simulink model "part1"  (R2021a)
settings: Solver=FixedStepDiscrete  StartTime=0  StopTime=20  FixedStep=0.1  RelTol=1e-3
values from neighbouring files (symbols this model uses):
  mu = [-2.06408447904 -1.49508472185]    [dataSet.mat]
  sig = [50.3880002876 29.2458553231]    [dataSet.mat]
undefined symbols (not defined in the file or in its folder): egoTargetSpd_kph
libraries: deeplib x2, fuzblock x1
settings Model: Creator=Ally  LastModifiedBy=Ally

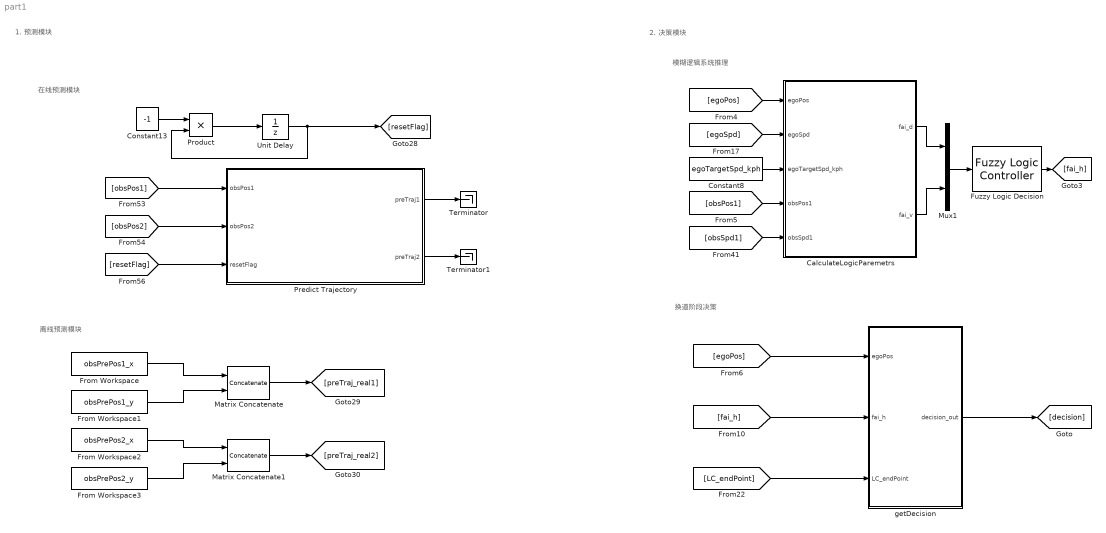
== system part1 ==
  note: 换道阶段决策
  note: 模糊逻辑系统推理
  note: 在线预测模块
  note: 离线预测模块
  note: 2. 决策模块
  note: 1. 预测模块
  CalculateLogicParemetrs : MATLAB Function  TreatAsAtomicUnit=on
  Constant13 : Constant  Value=-1
  Constant8 : Constant  Value=egoTargetSpd_kph
  From Workspace : FromWorkspace  VariableName=obsPrePos1_x
  From Workspace1 : FromWorkspace  VariableName=obsPrePos1_y
  From Workspace2 : FromWorkspace  VariableName=obsPrePos2_x
  From Workspace3 : FromWorkspace  VariableName=obsPrePos2_y
  Fuzzy Logic Decision : fuzblock/Fuzzy Logic  Controller  FIS='LCD.fis'  OutputSampleNumber=101  DataType=double  FuzzifiedInputs=off  RuleFiringStrengths=off  RuleOutputs=off  AggregatedOutputs=off  SimulateUsing=Interpreted execution  OutOfRangeInputValueMessage=warning  NoRuleFiredMessage=warning  EmptyOutputFuzzySetMessage=warning
  Matrix Concatenate : Concatenate  Mode=Multidimensional array  ConcatenateDimension=2
  Matrix Concatenate1 : Concatenate  Mode=Multidimensional array  ConcatenateDimension=2
  Mux1 : Mux  Inputs=2
  Predict Trajectory : Subsystem  TreatAsAtomicUnit=on
  Product : Product
  Terminator : Terminator
  Terminator1 : Terminator
  Unit Delay : UnitDelay  InitialCondition=1  SampleTime=-1  HasFrameUpgradeWarning=on
  getDecision : MATLAB Function  TreatAsAtomicUnit=on
  wires:
  CalculateLogicParemetrs/1(fai_d) -> Mux1/1
  [egoPos] -> CalculateLogicParemetrs/1(egoPos)
  getDecision/1(decision_out) -> [decision]
  CalculateLogicParemetrs/2(fai_v) -> Mux1/2
  [egoSpd] -> CalculateLogicParemetrs/2(egoSpd)
  [LC_endPoint] -> getDecision/3(LC_endPoint)
  Mux1/1 -> Fuzzy Logic Decision/1
  [egoPos] -> getDecision/1(egoPos)
  Constant8/1 -> CalculateLogicParemetrs/3(egoTargetSpd_kph)
  [obsPos1] -> CalculateLogicParemetrs/4(obsPos1)
  [obsSpd1] -> CalculateLogicParemetrs/5(obsSpd1)
  Product/1 -> Unit Delay/1
  Unit Delay/1 -> [resetFlag], Product/2
  Constant13/1 -> Product/1
  [resetFlag] -> Predict Trajectory/3(resetFlag)
  [obsPos1] -> Predict Trajectory/1(obsPos1)
  [obsPos2] -> Predict Trajectory/2(obsPos2)
  Predict Trajectory/1(preTraj1) -> Terminator/1
  Predict Trajectory/2(preTraj2) -> Terminator1/1
  From Workspace/1 -> Matrix Concatenate/1
  From Workspace1/1 -> Matrix Concatenate/2
  From Workspace2/1 -> Matrix Concatenate1/1
  From Workspace3/1 -> Matrix Concatenate1/2
  Matrix Concatenate/1 -> [preTraj_real1]
  Matrix Concatenate1/1 -> [preTraj_real2]
  Fuzzy Logic Decision/1 -> [fai_h]
  [fai_h] -> getDecision/2(fai_h)

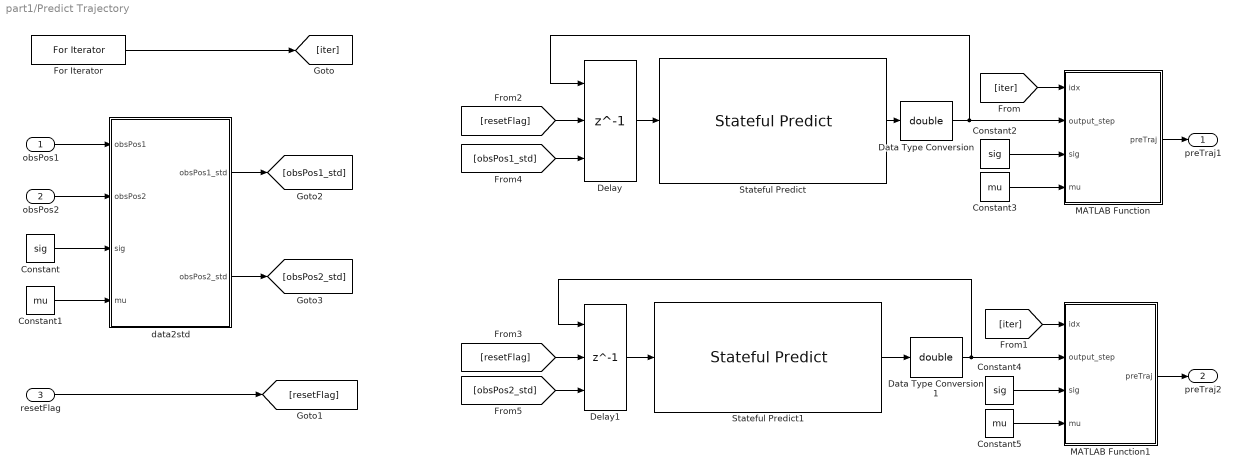
== system part1/Predict Trajectory ==
  obsPos1 : Inport
  obsPos2 : Inport  Port=2
  resetFlag : Inport  Port=3
  Constant : Constant  Value=sig
  Constant1 : Constant  Value=mu
  Constant2 : Constant  Value=sig
  Constant3 : Constant  Value=mu
  Constant4 : Constant  Value=sig
  Constant5 : Constant  Value=mu
  Data Type Conversion : DataTypeConversion  OutDataTypeStr=double
  Data Type Conversion1 : DataTypeConversion  OutDataTypeStr=double
  Delay : Delay  DelayLength=1  InitialConditionSource=Input port  ExternalReset=Either
      settings: InputPortMap=u0,r5,p4
  Delay1 : Delay  DelayLength=1  InitialConditionSource=Input port  ExternalReset=Either
      settings: InputPortMap=u0,r5,p4
  For Iterator : ForIterator  IterationLimit=80
  MATLAB Function : MATLAB Function  TreatAsAtomicUnit=on
  MATLAB Function1 : MATLAB Function  TreatAsAtomicUnit=on
  Stateful Predict : deeplib/Stateful Predict  Network=Network from MAT-file  NetworkFunction=untitled  NetworkFilePath=C:\Users\Ally\Desktop\LSTM.mat  InputDataFormats={ '', '' }  SampleTime=-1  ForceInterpretedSim=off  EnableDLNetwork=on
      settings: SourceProductBaseCode=NN
  Stateful Predict1 : deeplib/Stateful Predict  Network=Network from MAT-file  NetworkFunction=untitled  NetworkFilePath=C:\Users\Ally\Desktop\LSTM.mat  InputDataFormats={ '', '' }  SampleTime=-1  ForceInterpretedSim=off  EnableDLNetwork=on
      settings: SourceProductBaseCode=NN
  data2std : MATLAB Function  TreatAsAtomicUnit=on
  preTraj1 : Outport
  preTraj2 : Outport  Port=2
  wires:
  Delay/1 -> Stateful Predict/1
  Stateful Predict/1 -> Data Type Conversion/1
  Data Type Conversion/1 -> MATLAB Function/2(output_step), Delay/1
  Data Type Conversion1/1 -> MATLAB Function1/2(output_step), Delay1/1
  Stateful Predict1/1 -> Data Type Conversion1/1
  Delay1/1 -> Stateful Predict1/1
  For Iterator/1 -> [iter]
  [iter] -> MATLAB Function/1(idx)
  [iter] -> MATLAB Function1/1(idx)
  obsPos1/1 -> data2std/1(obsPos1)
  obsPos2/1 -> data2std/2(obsPos2)
  Constant1/1 -> data2std/4(mu)
  Constant/1 -> data2std/3(sig)
  Constant2/1 -> MATLAB Function/3(sig)
  Constant3/1 -> MATLAB Function/4(mu)
  resetFlag/1 -> [resetFlag]
  [resetFlag] -> Delay/2
  Constant5/1 -> MATLAB Function1/4(mu)
  Constant4/1 -> MATLAB Function1/3(sig)
  MATLAB Function/1(preTraj) -> preTraj1/1
  MATLAB Function1/1(preTraj) -> preTraj2/1
  [resetFlag] -> Delay1/2
  data2std/1(obsPos1_std) -> [obsPos1_std]
  [obsPos1_std] -> Delay/3
  data2std/2(obsPos2_std) -> [obsPos2_std]
  [obsPos2_std] -> Delay1/3

== matlab function part1/CalculateLogicParemetrs ==
  data: egoPos input; fai_d output; egoSpd input; egoTargetSpd_kph input; obsPos1 input; obsSpd1 input; fai_v output
function [fai_d,fai_v] = CalculateLogicParemetrs(egoPos,egoSpd,egoTargetSpd_kph, obsPos1, obsSpd1)
deltDist = sqrt((egoPos(1)-obsPos1(1))^2 + (egoPos(2)-obsPos1(2))^2);
egoSpd_abs = sqrt(egoSpd(1)^2 + egoSpd(2)^2);
obsSpd_abs = sqrt(obsSpd1(1)^2 + obsSpd1(2)^2);

% 计算安全距离模型
D_slf = (egoSpd_abs-obsSpd_abs)^2 / 2/(0.0524*egoSpd_abs-0.1215) + 0.8509*obsSpd_abs+1.6109;

% 计算车距期望系数
D_f = D_slf + 10;    % 车距期望值
if deltDist >= D_f
    fai_d = 1;
else
    fai_d = deltDist / D_f;
end

% 计算速度差值系数
egoTargetSpd_mps = egoTargetSpd_kph / 3.6;   
if egoSpd_abs >= egoTargetSpd_mps
    fai_v = 1;
else
    fai_v = (egoSpd_abs - obsSpd_abs) / egoTargetSpd_mps;
end

== matlab function part1/getDecision ==
  data: egoPos input; fai_h input; decision_out output; LC_endPoint input
function decision_out = getDecision(egoPos,fai_h,LC_endPoint)
persistent flag decision
if isempty(flag) || isempty(decision) 
    flag = 0;
    decision = 1;
end

if fai_h <= 0.5 && decision <= 1
    decision = 1;
else 
    % 计算本车位置与换道终点的距离
    dist = sqrt((egoPos(1) - LC_endPoint(1))^2 + (egoPos(2) - LC_endPoint(2))^2);
    if dist < 1 && flag == 0 || flag == 1
        decision = 3;
        flag = 1;
    else
        decision = 2;
    end
end
decision_out = decision;

== matlab function part1/Predict Trajectory/MATLAB Function ==
  data: idx input; preTraj output; output_step input; sig input; mu input
function preTraj = fcn(idx, output_step, sig, mu)
persistent output
if isempty(output)
    output = zeros(2,80);
end
for i = 1:2
    output(i,idx) = sig(i)*output_step(i,10) + mu(i);
    output(i,idx) = sig(i)*output_step(i,10) + mu(i);
end
preTraj = output;

== matlab function part1/Predict Trajectory/MATLAB Function1 ==
  data: idx input; preTraj output; output_step input; sig input; mu input
function preTraj = fcn(idx, output_step, sig, mu)
persistent output
if isempty(output)
    output = zeros(2,80);
end
for i = 1:2 
   output(i,idx) = sig(i)*output_step(i,10) + mu(i);
    output(i,idx) = sig(i)*output_step(i,10) + mu(i);
end
preTraj = output;

== matlab function part1/Predict Trajectory/data2std ==
  data: obsPos1 input; obsPos1_std output; obsPos2 input; obsPos2_std output; sig input; mu input
function [obsPos1_std, obsPos2_std] = data2std(obsPos1, obsPos2, sig, mu)
% 原始数据转为标准值数据
obsPos1_std = zeros(2,10);
obsPos2_std = zeros(2,10);
for i = 1:2
    obsPos1_std(i,:) = (obsPos1(i,:) - mu(i)) ./ sig(i);
    obsPos2_std(i,:) = (obsPos2(i,:) - mu(i)) ./ sig(i);
end
